simulink model "ADPthang8ban2"  (R2018b)
settings: Solver=ode3  StartTime=0.0  StopTime=20  FixedStep=0.00001  RelTol=1e-3
libraries: simulink x1
settings Model: Creator=User  LastModifiedBy=User

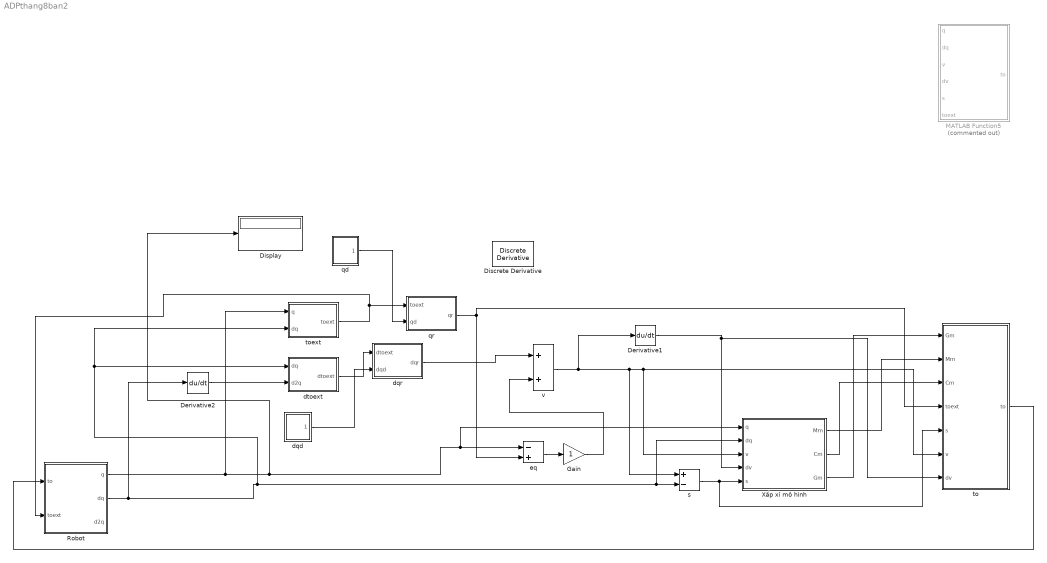
== system ADPthang8ban2 ==
  Derivative1 : Derivative
  Derivative2 : Derivative
  Discrete Derivative : simulink/Quick Insert/Discrete/Discrete Derivative  gainval=1.0  ICPrevScaledInput=0.0  OutMin=[]  OutMax=[]  OutDataType=fixdt(1, 16)  OutScaling=2^-10  DoSatur=off
      settings: SourceProductName=Simulink  SourceProductBaseCode=SL
  Display : Display
  Gain : Gain
  MATLAB Function5 : MATLAB Function  Commented=on  TreatAsAtomicUnit=on
  Robot : Subsystem
  Xấp xỉ mô hình : Subsystem
  dqd : Subsystem
  dqr : MATLAB Function  TreatAsAtomicUnit=on
  dtoext : MATLAB Function  TreatAsAtomicUnit=on
  eq : Sum  Inputs=-+
  qd : Subsystem
  qr : MATLAB Function  TreatAsAtomicUnit=on
  s : Sum  Inputs=+-
  to : MATLAB Function  TreatAsAtomicUnit=on
  toext : MATLAB Function  TreatAsAtomicUnit=on
  v : Sum
  wires:
  Robot/1(q) -> Display/1, Xấp xỉ mô hình/1(q), eq/1, toext/1(q)
  eq/1 -> Gain/1
  Gain/1 -> v/2
  toext/1(toext) -> Robot/2(toext), qr/1(toext)
  qd/1(Out1) -> qr/2(qd)
  dtoext/1(dtoext) -> dqr/1(dtoext)
  dqd/1(Out1) -> dqr/2(dqd)
  dqr/1(dqr) -> v/1
  qr/1(qr) -> to/4(toext), eq/2
  s/1 -> to/5(s), Xấp xỉ mô hình/5(s)
  Xấp xỉ mô hình/1(Mm) -> to/2(Mm)
  Xấp xỉ mô hình/3(Gm) -> to/1(Gm)
  Xấp xỉ mô hình/2(Cm) -> to/3(Cm)
  to/1(to) -> Robot/1(to)
  Derivative1/1 -> to/7(dv), Xấp xỉ mô hình/4(dv)
  v/1 -> to/6(v), Xấp xỉ mô hình/3(v), s/1, Derivative1/1
  Robot/2(dq) -> Derivative2/1, dtoext/1(dq), toext/2(dq), Xấp xỉ mô hình/2(dq), s/2
  Derivative2/1 -> dtoext/2(d2q)

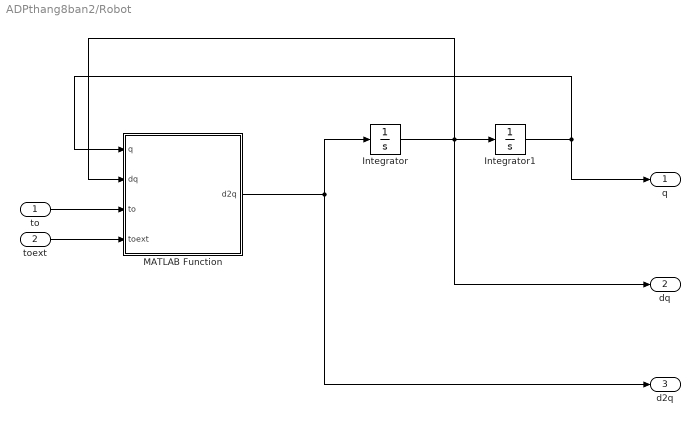
== system ADPthang8ban2/Robot ==
  to : Inport
  toext : Inport  Port=2
  Integrator : Integrator  InitialCondition=[0;0]
  Integrator1 : Integrator  InitialCondition=[2.6;-2.6]
  MATLAB Function : MATLAB Function  TreatAsAtomicUnit=on
  q : Outport
  dq : Outport  Port=2
  d2q : Outport  Port=3
  wires:
  Integrator1/1 -> q/1, MATLAB Function/1(q)
  Integrator/1 -> dq/1, Integrator1/1, MATLAB Function/2(dq)
  to/1 -> MATLAB Function/3(to)
  toext/1 -> MATLAB Function/4(toext)
  MATLAB Function/1(d2q) -> d2q/1, Integrator/1

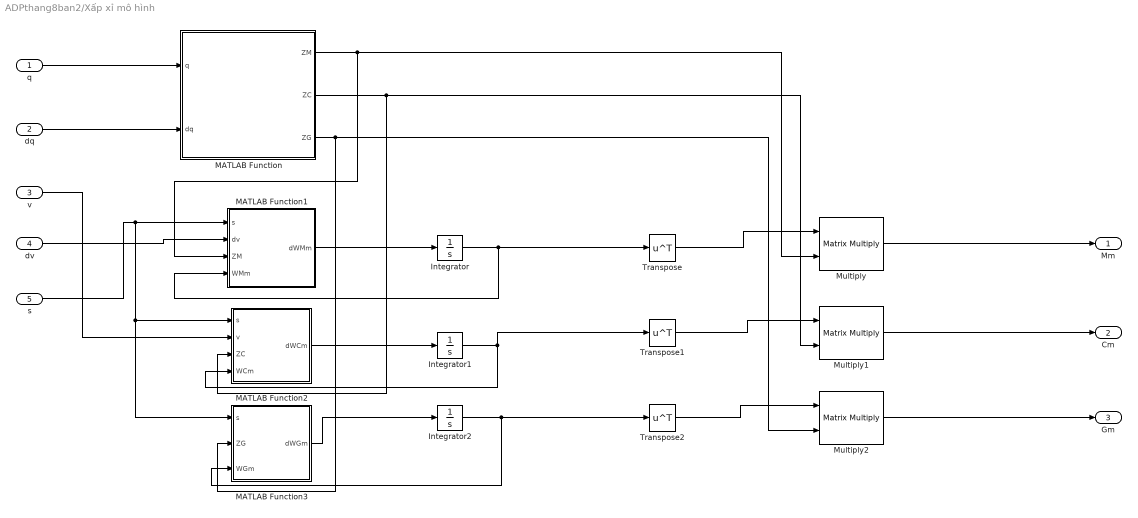
== system ADPthang8ban2/Xấp xỉ mô hình ==
  q : Inport
  dq : Inport  Port=2
  v : Inport  Port=3
  dv : Inport  Port=4
  s : Inport  Port=5
  Integrator : Integrator  InitialCondition=zeros(162,2)
  Integrator1 : Integrator  InitialCondition=zeros(324,2)
  Integrator2 : Integrator  InitialCondition=zeros(81,2)
  MATLAB Function : MATLAB Function  TreatAsAtomicUnit=on
  MATLAB Function1 : MATLAB Function  TreatAsAtomicUnit=on
  MATLAB Function2 : MATLAB Function  TreatAsAtomicUnit=on
  MATLAB Function3 : MATLAB Function  TreatAsAtomicUnit=on
  Multiply : Product  Multiplication=Matrix(*)
  Multiply1 : Product  Multiplication=Matrix(*)
  Multiply2 : Product  Multiplication=Matrix(*)
  Transpose : Math  Operator=transpose  SaturateOnIntegerOverflow=on
  Transpose1 : Math  Operator=transpose  SaturateOnIntegerOverflow=on
  Transpose2 : Math  Operator=transpose  SaturateOnIntegerOverflow=on
  Mm : Outport
  Cm : Outport  Port=2
  Gm : Outport  Port=3
  wires:
  q/1 -> MATLAB Function/1(q)
  dq/1 -> MATLAB Function/2(dq)
  MATLAB Function/1(ZM) -> MATLAB Function1/3(ZM), Multiply/2
  MATLAB Function/2(ZC) -> MATLAB Function2/3(ZC), Multiply1/2
  MATLAB Function/3(ZG) -> MATLAB Function3/2(ZG), Multiply2/2
  Integrator/1 -> MATLAB Function1/4(WMm), Transpose/1
  Integrator1/1 -> Transpose1/1, MATLAB Function2/4(WCm)
  Integrator2/1 -> MATLAB Function3/3(WGm), Transpose2/1
  Transpose/1 -> Multiply/1
  Transpose1/1 -> Multiply1/1
  Transpose2/1 -> Multiply2/1
  Multiply/1 -> Mm/1
  Multiply1/1 -> Cm/1
  Multiply2/1 -> Gm/1
  s/1 -> MATLAB Function3/1(s), MATLAB Function2/1(s), MATLAB Function1/1(s)
  dv/1 -> MATLAB Function1/2(dv)
  MATLAB Function1/1(dWMm) -> Integrator/1
  MATLAB Function2/1(dWCm) -> Integrator1/1
  v/1 -> MATLAB Function2/2(v)
  MATLAB Function3/1(dWGm) -> Integrator2/1

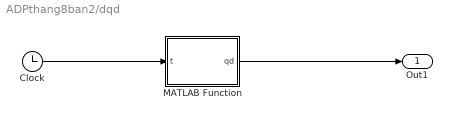
== system ADPthang8ban2/dqd ==
  Clock : Clock
  MATLAB Function : MATLAB Function  TreatAsAtomicUnit=on
  Out1 : Outport
  wires:
  MATLAB Function/1(qd) -> Out1/1
  Clock/1 -> MATLAB Function/1(t)

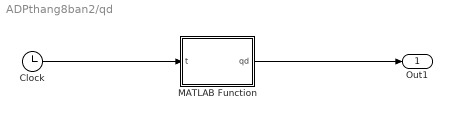
== system ADPthang8ban2/qd ==
  Clock : Clock
  MATLAB Function : MATLAB Function  TreatAsAtomicUnit=on
  Out1 : Outport
  wires:
  Clock/1 -> MATLAB Function/1(t)
  MATLAB Function/1(qd) -> Out1/1

== matlab function ADPthang8ban2/toext ==
  data: q input; toext output; dq input
function toext = fcn(q,dq)
toext=-0.01*dq-(q-0.3);
end

== matlab function ADPthang8ban2/Robot/MATLAB Function ==
  data: q input; d2q output; dq input; to input; toext input
function d2q  = fcn(q,dq,to,toext)
m1=2;
m2=2;
l1=0.2;
l2=0.2;
J1=0.027;
J2=0.027;
q2=q(2);
q1=q(1);
M11=J1+J2+m1*l1^2/4+m2*l2^2/4+m2*l1^2+m2*l1*l2*cos(q2);
M12=J2+m2*l2^2/4+m2*l1*l2/2*cos(q2);
M21=M12;
M22=J2+m2*l2^2/4;
M=[M11 M12;M21 M22];
dq1=dq(1);
dq2=dq(2);
C11=-m2*l1*l2/2*sin(q2)*dq2;
C12=-m2*l1*l2/2*sin(q2)*(dq1+dq2);
C21=m1*l1*l2/2*sin(q2)*dq1;
C=[C11 C12;C21 0];
g=9.8;
G1=m1*g*l1/2*cos(q1)+m2*g*(l1*cos(q1)+l2/2*cos(q1+q2));
G2=m2*g*l2/2*cos(q1+q2);
G=[G1;G2];
d2q=M\(to-toext-C*dq-G);
end

== matlab function ADPthang8ban2/qr ==
  data: toext input; qr output; qd input
function qr = fcn(toext,qd)
qr=(toext+0.7021*(qd-0.3))/0.4142+0.3;

== matlab function ADPthang8ban2/qd/MATLAB Function ==
  data: t input; qd output
function qd = fcn(t)
qd=[0.5-0.2*exp(-t);
    0.3-0.3*exp(-t)];
end

== matlab function ADPthang8ban2/to ==
  data: Gm input; to output; Mm input; Cm input; toext input; s input; v input; dv input
function to = fcn(Gm,Mm,Cm,toext,s,v,dv)
K=[1.2 0;0 1.2];
to=Gm+Mm*dv+Cm*v+toext+K*s;
end

== matlab function ADPthang8ban2/dqd/MATLAB Function ==
  data: t input; qd output
function qd = fcn(t)
qd=[0.2*exp(-t);
    0.3*exp(-t)];
end

== matlab function ADPthang8ban2/dtoext ==
  data: dq input; d2q input; dtoext output
function dtoext = fcn(dq,d2q)
dtoext=-0.01*d2q-(dq);
end

== matlab function ADPthang8ban2/dqr ==
  data: dtoext input; dqr output; dqd input
function dqr = fcn(dtoext,dqd)
dqr=(dtoext+0.7021*(dqd))/0.4142;

== matlab function ADPthang8ban2/MATLAB Function5 ==
  data: q input; to output; dq input; v input; dv input; s input; toext input
function to = fcn(q,dq,v,dv,s,toext)
m1=2;
m2=2;
l1=0.2;
l2=0.2;
J1=0.027;
J2=0.027;
q2=q(2);
q1=q(1);
M11=J1+J2+m1*l1^2/4+m2*l2^2/4+m2*l1^2+m2*l1*l2*cos(q2);
M12=J2+m2*l2^2/4+m2*l1*l2/2*cos(q2);
M21=M12;
M22=J2+m2*l2^2/4;
M=[M11 M12;M21 M22];
dq1=dq(1);
dq2=dq(2);
C11=-m2*l1*l2/2*sin(q2)*dq2;
C12=-m2*l1*l2/2*sin(q2)*(dq1+dq2);
C21=m1*l1*l2/2*sin(q2)*dq1;
C=[C11 C12;C21 0];
g=9.8;
G1=m1*g*l1/2*cos(q1)+m2*g*(l1*cos(q1)+l2/2*cos(q1+q2));
G2=m2*g*l2/2*cos(q1+q2);
G=[G1;G2];
K=[1.2 0;0 1.2];
to=G+M*dv+C*v+toext+K*s;
end

== matlab function ADPthang8ban2/Xấp xỉ mô hình/MATLAB Function2 ==
  data: s input; v input; ZC input; WCm input; dWCm output
function dWCm= fcn(s,v,ZC,WCm)
QC=0.1;
sC=0;
dWCm=-1/QC*(ZC*v*s'+sC*WCm);
end

== matlab function ADPthang8ban2/Xấp xỉ mô hình/MATLAB Function3 ==
  data: s input; ZG input; WGm input; dWGm output
function dWGm = fcn(s,ZG,WGm)
QG=0.1;
sG=0;
dWGm=-1/QG*(ZG*s'+sG*WGm);
end

== matlab function ADPthang8ban2/Xấp xỉ mô hình/MATLAB Function ==
  data: q input; ZM output; dq input; ZC output; ZG output
function [ZM,ZC,ZG] = fcn(q,dq)
qi=[ -3.0000   -3.0000
   -3.0000   -2.0000
   -3.0000   -1.0000
   -3.0000   -0.5000
   -3.0000         0
   -3.0000    0.5000
   -3.0000    1.0000
   -3.0000    2.0000
   -3.0000    3.0000
   -2.0000   -3.0000
   -2.0000   -2.0000
   -2.0000   -1.0000
   -2.0000   -0.5000
   -2.0000         0
   -2.0000    0.5000
   -2.0000    1.0000
   -2.0000    2.0000
   -2.0000    3.0000
   -1.0000   -3.0000
   -1.0000   -2.0000
   -1.0000   -1.0000
   -1.0000   -0.5000
   -1.0000         0
   -1.0000    0.5000
   -1.0000    1.0000
   -1.0000    2.0000
   -1.0000    3.0000
   -0.5000   -3.0000
   -0.5000   -2.0000
   -0.5000   -1.0000
   -0.5000   -0.5000
   -0.5000         0
   -0.5000    0.5000
   -0.5000    1.0000
   -0.5000    2.0000
   -0.5000    3.0000
         0   -3.0000
         0   -2.0000
         0   -1.0000
         0   -0.5000
         0         0
         0    0.5000
         0    1.0000
         0    2.0000
         0    3.0000
    0.5000   -3.0000
    0.5000   -2.0000
    0.5000   -1.0000
    0.5000   -0.5000
    0.5000         0
    0.5000    0.5000
    0.5000    1.0000
    0.5000    2.0000
    0.5000    3.0000
    1.0000   -3.0000
    1.0000   -2.0000
    1.0000   -1.0000
    1.0000   -0.5000
    1.0000         0
    1.0000    0.5000
    1.0000    1.0000
    1.0000    2.0000
    1.0000    3.0000
    2.0000   -3.0000
    2.0000   -2.0000
    2.0000   -1.0000
    2.0000   -0.5000
    2.0000         0
    2.0000    0.5000
    2.0000    1.0000
    2.0000    2.0000
    2.0000    3.0000
    3.0000   -3.0000
    3.0000   -2.0000
    3.0000   -1.0000
    3.0000   -0.5000
    3.0000         0
    3.0000    0.5000
    3.0000    1.0000
    3.0000    2.0000
    3.0000    3.0000]';
dqi=qi;
Zq=zeros(81,1);
Zdq=zeros(81,1);
for i=1:81
    Zq(i)=exp(-(q-qi(:,i))'*(q-qi(:,i))/0.5^2);
    Zdq(i)=exp(-(dq-dqi(:,i))'*(dq-dqi(:,i))/0.5^2);
end
ZM=blkdiag(Zq,Zq);
ZC=blkdiag([Zq;Zdq],[Zq;Zdq]);
ZG=Zq;
end

== matlab function ADPthang8ban2/Xấp xỉ mô hình/MATLAB Function1 ==
  data: s input; dWMm output; dv input; ZM input; WMm input
function dWMm = fcn(s,dv,ZM,WMm)
QM=0.1;
sM=0;
dWMm=-1/QM*(ZM*dv*s'+sM*WMm);
end
